simulink model "Compare_Simscape_Simulink"  (R2023a)
settings: Solver=VariableStepAuto  StartTime=0.0  StopTime=10  RelTol=1e-3
model workspace (MAT data in the model file):
  Ks = 16000
  Kt = 190000
  Mb = 300
  Mb_max = 0.00266666666667
  Mb_min = 0.00392156862745
  Mw = 60
  Mw_max = 63
  Mw_min = 57
  bs_max = 1350
  bs_min = 650
  ks_max = 20800
  ks_min = 11200
  kt_max = 209000
  kt_min = 171000
values from neighbouring files (symbols this model uses):
  Ac = (inv(value(N)))*(value(A_hat) - value(Y)*A*value(X)-value(N)*Bc*C1*value(X)-value(Y)*B1*Cc*value(M)')*(inv(value(M)'))    [Active_suspension_output_FB.m]
  Bc = (inv(value(N)))* value(B_hat)    [Active_suspension_output_FB.m]
  bs = 1000    [Active_suspension_output_FB.m]
  Cc = value(C_hat)*(inv(value(M)'))    [Active_suspension_output_FB.m]
  ks = 16000    [Active_suspension_output_FB.m]
undefined symbols (not defined in the file or in its folder): K
libraries: fl_lib x22, nesl_utility x19, slpidlib x2, sdl_lib x2, spsStairGeneratorLib x1
settings Model: Creator=poke  LastModifiedBy=poke
settings OptimizationCC: ReuseModelBlockBuffer=off

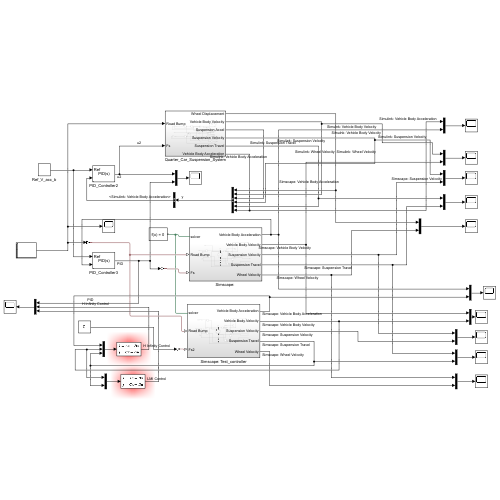
[thumbnail: Simulink's stored preview of the top-level diagram]
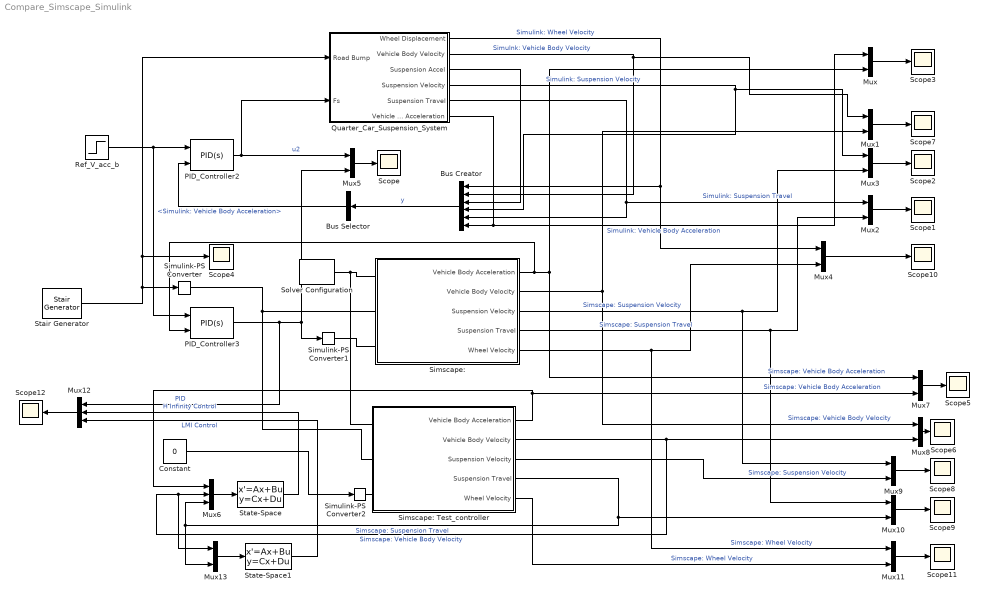
== system Compare_Simscape_Simulink ==
  Bus Creator : BusCreator  Inputs=6
  Bus Selector : BusSelector  OutputSignals=Simulink: Vehicle Body Acceleration
  Constant : Constant  Value=0
  Mux{,1..5,7..11,13} (12 alike) : Mux  Inputs=2
  Mux12 : Mux  Inputs=3
  Mux6 : Mux  Inputs=3
  PID_Controller2 : slpidlib/PID Controller (2DOF)  Controller=PID  Form=Parallel  TimeDomain=Continuous-time  UseExternalTs=off  SampleTime=-1  IntegratorMethod=Forward Euler  FilterMethod=Forward Euler  ControllerParametersSource=internal  P=10738.4637303228  I=251871.072818037  UseKiTs=off  D=98.7205538071968  N=3940.78612428139  UseFilter=on  b=0.0124821033791995  c=1.67293570854955e-05  TunerSelectOption=Transfer Function Based (PID Tuner App)  InitialConditionSource=internal  InitialConditionForIntegrator=0  InitialConditionForFilter=0  DifferentiatorICPrevScaledInput=0  ExternalReset=none  TrackingMode=off  Kt=1  LimitOutput=off  SatLimitsSource=internal  UpperSaturationLimit=inf  LowerSaturationLimit=-inf  LinearizeAsGain=on  AntiWindupMode=none  Kb=1  LimitIntegrator=off  UpperIntegratorSaturationLimit=inf  LowerIntegratorSaturationLimit=-inf  POutMin=[]  POutMax=[]  IOutMin=[]  IOutMax=[]  DOutMin=[]  DOutMax=[]  NOutMin=[]  NOutMax=[]  bOutMin=[]  bOutMax=[]  cOutMin=[]  cOutMax=[]  SumOutMin=[]  SumOutMax=[]  SaturationOutMin=[]  SaturationOutMax=[]  PParamMin=[]  PParamMax=[]  IParamMin=[]  IParamMax=[]  DParamMin=[]  DParamMax=[]  NParamMin=[]  NParamMax=[]  bParamMin=[]  bParamMax=[]  cParamMin=[]  cParamMax=[]  KbParamMin=[]  KbParamMax=[]  KtParamMin=[]  KtParamMax=[]  KbOutMin=[]  KbOutMax=[]  KtOutMin=[]  KtOutMax=[]  IntegratorOutMin=[]  IntegratorOutMax=[]  FilterOutMin=[]  FilterOutMax=[]  SumI1OutMin=[]  SumI1OutMax=[]  SumI2OutMin=[]  SumI2OutMax=[]  SumI3OutMin=[]  SumI3OutMax=[]  SumI4OutMin=[]  SumI4OutMax=[]  SumDOutMin=[]  SumDOutMax=[]  Sum1OutMin=[]  Sum1OutMax=[]  Sum2OutMin=[]  Sum2OutMax=[]  Sum3OutMin=[]  Sum3OutMax=[]  DifferentiatorOutMin=[]  DifferentiatorOutMax=[]  FilterDiffOutCoefMin=[]  FilterDiffOutCoefMax=[]  ReciprocalOutMin=[]  ReciprocalOutMax=[]  SumDenOutMin=[]  SumDenOutMax=[]  SumNumOutMin=[]  SumNumOutMax=[]  DivideOutMin=[]  DivideOutMax=[]  UdiffTsProdOutMin=[]  UdiffTsProdOutMax=[]  NTsProdOutMin=[]  NTsProdOutMax=[]  UintegralTsProdOutMin=[]  UintegralTsProdOutMax=[]  UngainTsProdOutMin=[]  UngainTsProdOutMax=[]  ClampingZeroOutDataTypeStr=Inherit: Inherit via back propagation  ClampingZeroOutMin=[]  ClampingZeroOutMax=[]  FilterDenConstantOutDataTypeStr=Inherit: Inherit via back propagation  FilterDenConstantOutMin=[]  FilterDenConstantOutMax=[]  PCopyOutDataTypeStr=Inherit: Inherit via back propagation  PCopyOutMin=[]  PCopyOutMax=[]  NCopyOutDataTypeStr=Inherit: Inherit via back propagation  NCopyOutMin=[]  NCopyOutMax=[]  IntegratorContinuousStateAttributes=''  IntegratorStateMustResolveToSignalObject=off  IntegratorRTWStateStorageClass=Auto  FilterContinuousStateAttributes=''  FilterStateMustResolveToSignalObject=off  FilterRTWStateStorageClass=Auto  ParallelPVariant=InternalParameters  IdealPVariant=Disabled  IVariant=InternalParameters  DVariant=InternalParameters  bVariant=InternalParameters  cVariant=InternalParameters  IntegratorVariant=Continuous  SatVariant=Disabled  AWVariant=Passthrough  PCopyVariant=Disabled  TRVariant=Disabled  FdbkBlocksVariant=Forward  IdealPFdbkVariant=Disabled  SatFdbkVariant=Disabled  DerivativeFilterVariant=ContFilter  NVariant=InternalParameters  NCopyVariant=Disabled  FilterICVariant=InternalICsFilter  IntegratorICVariant=InternalICs  ExternalResetVariant=Disabled  TRSumVariant=Passthrough  SumFdbkVariant=Disabled  SumVariant=Sum_PID  TsampFilterVariant=InternalTs  TsampNgainVariant=Passthrough  TsampIntegralVariant=Disabled_SignalSpec  ExternalSaturationOutDataTypeStr=Inherit: Same as second input
  PID_Controller3 : slpidlib/PID Controller (2DOF)  Controller=PID  Form=Parallel  TimeDomain=Continuous-time  UseExternalTs=off  SampleTime=-1  IntegratorMethod=Forward Euler  FilterMethod=Forward Euler  ControllerParametersSource=internal  P=10738.4637303228  I=251871.072818037  UseKiTs=off  D=98.7205538071968  N=3940.78612428139  UseFilter=on  b=0.0124821033791995  c=1.67293570854955e-05  TunerSelectOption=Transfer Function Based (PID Tuner App)  InitialConditionSource=internal  InitialConditionForIntegrator=0  InitialConditionForFilter=0  DifferentiatorICPrevScaledInput=0  ExternalReset=none  TrackingMode=off  Kt=1  LimitOutput=off  SatLimitsSource=internal  UpperSaturationLimit=inf  LowerSaturationLimit=-inf  LinearizeAsGain=on  AntiWindupMode=none  Kb=1  LimitIntegrator=off  UpperIntegratorSaturationLimit=inf  LowerIntegratorSaturationLimit=-inf  POutMin=[]  POutMax=[]  IOutMin=[]  IOutMax=[]  DOutMin=[]  DOutMax=[]  NOutMin=[]  NOutMax=[]  bOutMin=[]  bOutMax=[]  cOutMin=[]  cOutMax=[]  SumOutMin=[]  SumOutMax=[]  SaturationOutMin=[]  SaturationOutMax=[]  PParamMin=[]  PParamMax=[]  IParamMin=[]  IParamMax=[]  DParamMin=[]  DParamMax=[]  NParamMin=[]  NParamMax=[]  bParamMin=[]  bParamMax=[]  cParamMin=[]  cParamMax=[]  KbParamMin=[]  KbParamMax=[]  KtParamMin=[]  KtParamMax=[]  KbOutMin=[]  KbOutMax=[]  KtOutMin=[]  KtOutMax=[]  IntegratorOutMin=[]  IntegratorOutMax=[]  FilterOutMin=[]  FilterOutMax=[]  SumI1OutMin=[]  SumI1OutMax=[]  SumI2OutMin=[]  SumI2OutMax=[]  SumI3OutMin=[]  SumI3OutMax=[]  SumI4OutMin=[]  SumI4OutMax=[]  SumDOutMin=[]  SumDOutMax=[]  Sum1OutMin=[]  Sum1OutMax=[]  Sum2OutMin=[]  Sum2OutMax=[]  Sum3OutMin=[]  Sum3OutMax=[]  DifferentiatorOutMin=[]  DifferentiatorOutMax=[]  FilterDiffOutCoefMin=[]  FilterDiffOutCoefMax=[]  ReciprocalOutMin=[]  ReciprocalOutMax=[]  SumDenOutMin=[]  SumDenOutMax=[]  SumNumOutMin=[]  SumNumOutMax=[]  DivideOutMin=[]  DivideOutMax=[]  UdiffTsProdOutMin=[]  UdiffTsProdOutMax=[]  NTsProdOutMin=[]  NTsProdOutMax=[]  UintegralTsProdOutMin=[]  UintegralTsProdOutMax=[]  UngainTsProdOutMin=[]  UngainTsProdOutMax=[]  ClampingZeroOutDataTypeStr=Inherit: Inherit via back propagation  ClampingZeroOutMin=[]  ClampingZeroOutMax=[]  FilterDenConstantOutDataTypeStr=Inherit: Inherit via back propagation  FilterDenConstantOutMin=[]  FilterDenConstantOutMax=[]  PCopyOutDataTypeStr=Inherit: Inherit via back propagation  PCopyOutMin=[]  PCopyOutMax=[]  NCopyOutDataTypeStr=Inherit: Inherit via back propagation  NCopyOutMin=[]  NCopyOutMax=[]  IntegratorContinuousStateAttributes=''  IntegratorStateMustResolveToSignalObject=off  IntegratorRTWStateStorageClass=Auto  FilterContinuousStateAttributes=''  FilterStateMustResolveToSignalObject=off  FilterRTWStateStorageClass=Auto  ParallelPVariant=InternalParameters  IdealPVariant=Disabled  IVariant=InternalParameters  DVariant=InternalParameters  bVariant=InternalParameters  cVariant=InternalParameters  IntegratorVariant=Continuous  SatVariant=Disabled  AWVariant=Passthrough  PCopyVariant=Disabled  TRVariant=Disabled  FdbkBlocksVariant=Forward  IdealPFdbkVariant=Disabled  SatFdbkVariant=Disabled  DerivativeFilterVariant=ContFilter  NVariant=InternalParameters  NCopyVariant=Disabled  FilterICVariant=InternalICsFilter  IntegratorICVariant=InternalICs  ExternalResetVariant=Disabled  TRSumVariant=Passthrough  SumFdbkVariant=Disabled  SumVariant=Sum_PID  TsampFilterVariant=InternalTs  TsampNgainVariant=Passthrough  TsampIntegralVariant=Disabled_SignalSpec  ExternalSaturationOutDataTypeStr=Inherit: Same as second input
  Quarter_Car_Suspension_System : Subsystem
  Ref_V_acc_b : Step  After=0  SampleTime=0
  Scope{,1..12} (13 alike) : Scope
  "Simscape: " : Subsystem
  Simscape: Test_controller : Subsystem
  Simulink-PS Converter : nesl_utility/Simulink-PS Converter  PhysicalDomain=network_engine_domain  SubClassName=ps_input  LeftPortType=input  RightPortType=output  PseudoPeriodic=off  Frequencies=[]  NoiseDistribution=none  NoiseParameters=[]  Unit=1  AffineConversion=off  FilteringAndDerivatives=provide  SimscapeFilterOrder=1  InputFilterTimeConstant=0.001  UdotUserProvided=0
  Simulink-PS Converter1 : nesl_utility/Simulink-PS Converter  PhysicalDomain=network_engine_domain  SubClassName=ps_input  LeftPortType=input  RightPortType=output  PseudoPeriodic=off  Frequencies=[]  NoiseDistribution=none  NoiseParameters=[]  Unit=1  AffineConversion=off  FilteringAndDerivatives=provide  SimscapeFilterOrder=1  InputFilterTimeConstant=0.001  UdotUserProvided=0
  Simulink-PS Converter2 : nesl_utility/Simulink-PS Converter  PhysicalDomain=network_engine_domain  SubClassName=ps_input  LeftPortType=input  RightPortType=output  PseudoPeriodic=off  Frequencies=[]  NoiseDistribution=none  NoiseParameters=[]  Unit=1  AffineConversion=off  FilteringAndDerivatives=provide  SimscapeFilterOrder=1  InputFilterTimeConstant=0.001  UdotUserProvided=0
  Solver Configuration : nesl_utility/Solver Configuration  PhysicalDomain=network_engine_domain  SubClassName=solver  LeftPortType=input  RightPortType=generic  Tones=[]  Harmonics=[]  SimulateNoise=off  Profile=off  UseLocalSampling=off  EnableSwitchedLinearOptims=on  FrequencyDomain=off  UseCCode=off  RelTol=0.001  AbsTol=0.001  MinStep=1e-09  ToWorkspace=off  RevertToSquareIcSolve=off  NumHomotopyIterations=100  PhasorMode=off  PhasorModeNumHarmonics=1  ConsistencySolver=NEWTON_XTOL_AFTER_FTOL  IndexReductionMethod=DerivativeReplacement  DoDC=off  ResidualTolerance=1e-09  ConsistencyTolSource=GLOBAL  ConsistencyAbsTol=0.001  ConsistencyRelTol=0.001  ConsistencyTolFactor=0.001  UseLocalSolver=off  LocalSolverChoice=NE_BACKWARD_EULER_ADVANCER  ResolveIndetEquations=on  FunctionEvalNumThread=1  LocalSolverSampleTime=0.001  DoFixedCost=off  MaxNonlinIter=3  MaxModeIter=2  ComputeImpulses=off  ImpulseIterations=2  LinearAlgebra=auto  LinearAlgebraNumThread=0  EquationFormulation=NE_TIME_EF  DelaysMemoryBudget=1024  AutomaticFiltering=on  FilteringTimeConstant=0.001  PartitionStorageMethod=AS_NEEDED  PartitionMemoryBudget=1024  PartitionMethod=ROBUST
  Stair Generator : spsStairGeneratorLib/Stair Generator  t=t  e=roaddist  Ts=0
  State-Space : StateSpace  A=K.A  B=K.B  C=K.C  D=K.D  InitialCondition=0
  State-Space1 : StateSpace  A=Ac  B=Bc  C=Cc  D=[0 0]  InitialCondition=0
  wires:
  Quarter_Car_Suspension_System/6(Vehicle Body Acceleration) -> Mux/1, Bus Creator/6  "Simulink: Vehicle Body Acceleration"
  Quarter_Car_Suspension_System/4(Suspension Velocity) -> Bus Creator/4, Mux3/1  "Simulink: Suspension Velocity"
  Quarter_Car_Suspension_System/1(Wheel Displacement) -> Bus Creator/1, Mux4/1  "Simulink: Wheel Velocity"
  Quarter_Car_Suspension_System/2(Vehicle Body Velocity) -> Bus Creator/2, Mux1/1  "Simulnk: Vehicle Body Velocity"
  Mux/1 -> Scope3/1
  Mux1/1 -> Scope7/1
  Quarter_Car_Suspension_System/5(Suspension Travel) -> Bus Creator/5, Mux2/1  "Simulink: Suspension Travel"
  Mux2/1 -> Scope1/1
  Mux3/1 -> Scope2/1
  Mux4/1 -> Scope10/1
  "Simscape: "/1(Vehicle Body Acceleration) -> PID_Controller3/2, Mux7/1, Mux/2  "Simscape: Vehicle Body Acceleration"
  "Simscape: "/2(Vehicle Body Velocity) -> Mux8/1, Mux1/2  "Simscape: Vehicle Body Velocity"
  "Simscape: "/3(Suspension Velocity) -> Mux9/1, Mux3/2  "Simscape: Suspension Velocity"
  "Simscape: "/4(Suspension Travel) -> Mux10/1, Mux2/2  "Simscape: Suspension Travel"
  "Simscape: "/5(Wheel Velocity) -> Mux11/1, Mux4/2  "Simscape: Wheel Velocity"
  PID_Controller2/1 -> Mux5/1, Quarter_Car_Suspension_System/2(Fs)  "u2"
  Bus Selector/1 -> PID_Controller2/2  "<Simulink: Vehicle Body Acceleration>"
  Bus Creator/1 -> Bus Selector/1  "y"
  Ref_V_acc_b/1 -> PID_Controller3/1, PID_Controller2/1
  Quarter_Car_Suspension_System/3(Suspension Accel) -> Bus Creator/3
  Stair Generator/1 -> Scope4/1, Quarter_Car_Suspension_System/1(Road Bump), Simulink-PS Converter/1
  PID_Controller3/1 -> Mux12/1, Simulink-PS Converter1/1, Mux5/2  "PID"
  Mux5/1 -> Scope/1
  State-Space/1 -> Mux12/2  "H Infinity Control"
  Mux6/1 -> State-Space/1
  Simscape: Test_controller/1(Vehicle Body Acceleration) -> Mux7/2, Mux6/1  "Simscape: Vehicle Body Acceleration"
  Simscape: Test_controller/2(Vehicle Body Velocity) -> Mux8/2, Mux13/1, Mux6/2  "Simscape: Vehicle Body Velocity"
  Simscape: Test_controller/5(Wheel Velocity) -> Mux11/2  "Simscape: Wheel Velocity"
  Mux7/1 -> Scope5/1
  Mux8/1 -> Scope6/1
  Mux9/1 -> Scope8/1
  Simscape: Test_controller/3(Suspension Velocity) -> Mux9/2  "Simscape: Suspension Velocity"
  Mux10/1 -> Scope9/1
  Simscape: Test_controller/4(Suspension Travel) -> Mux6/3, Mux13/2, Mux10/2  "Simscape: Suspension Travel"
  Mux11/1 -> Scope11/1
  Mux12/1 -> Scope12/1
  Mux13/1 -> State-Space1/1
  State-Space1/1 -> Mux12/3  "LMI Control"
  Constant/1 -> Simulink-PS Converter2/1
  connections:
  Simulink-PS Converter/RConn1 -- Simscape: Test_controller/LConn2 -- "Simscape: "/LConn2
  Simulink-PS Converter1/RConn1 -- "Simscape: "/LConn3
  Simulink-PS Converter2/RConn1 -- Simscape: Test_controller/LConn3
  Solver Configuration/RConn1 -- Simscape: Test_controller/LConn1 -- "Simscape: "/LConn1

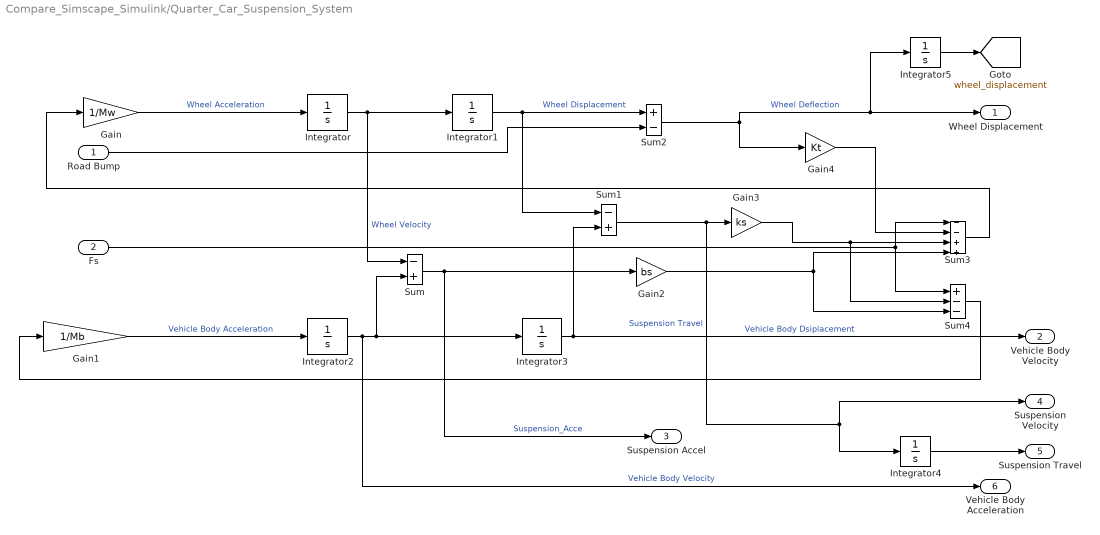
== system Compare_Simscape_Simulink/Quarter_Car_Suspension_System ==
  Road Bump : Inport
  Fs : Inport  Port=2
  Gain : Gain  Gain=1/Mw  ParamMin=1/Mw_max  ParamMax=1/Mw_min
  Gain1 : Gain  Gain=1/Mb  ParamMin=Mb_max  ParamMax=Mb_min
  Gain2 : Gain  Gain=bs  ParamMin=bs_min  ParamMax=bs_max
  Gain3 : Gain  Gain=ks  ParamMin=ks_min  ParamMax=ks_max
  Gain4 : Gain  Gain=Kt  ParamMin=kt_min  ParamMax=kt_max
  Integrator{,1..5} (6 alike) : Integrator
  Sum : Sum  Inputs=-+
  Sum1 : Sum  Inputs=-+
  Sum2 : Sum  Inputs=+-
  Sum3 : Sum  Inputs=--++
  Sum4 : Sum  Inputs=+--
  Wheel Displacement : Outport
  Vehicle Body Velocity : Outport  Port=2
  Suspension Accel : Outport  Port=3
  Suspension Velocity : Outport  Port=4
  Suspension Travel : Outport  Port=5
  Vehicle Body Acceleration : Outport  Port=6
  tag scope: wheel_displacement=global
  wires:
  Gain/1 -> Integrator/1  "Wheel Acceleration"
  Gain2/1 -> Sum4/3, Sum3/4
  Sum4/1 -> Gain1/1
  Gain1/1 -> Integrator2/1  "Vehicle Body Acceleration"
  Sum2/1 -> Gain4/1, Integrator5/1, Wheel Displacement/1  "Wheel Deflection"
  Sum3/1 -> Gain/1
  Sum/1 -> Suspension Accel/1, Gain2/1  "Suspension_Acce"
  Integrator2/1 -> Vehicle Body Acceleration/1, Integrator3/1, Sum/2  "Vehicle Body Velocity"
  Integrator1/1 -> Sum2/1, Sum1/1  "Wheel Displacement"
  Integrator3/1 -> Vehicle Body Velocity/1, Sum1/2  "Vehicle Body Dsiplacement"
  Integrator/1 -> Integrator1/1, Sum/1  "Wheel Velocity"
  Gain3/1 -> Sum4/2, Sum3/3
  Road Bump/1 -> Sum2/2
  Sum1/1 -> Suspension Velocity/1, Integrator4/1, Gain3/1  "Suspension Travel"
  Gain4/1 -> Sum3/2
  Integrator4/1 -> Suspension Travel/1
  Integrator5/1 -> [wheel_displacement]
  Fs/1 -> Sum4/1, Sum3/1

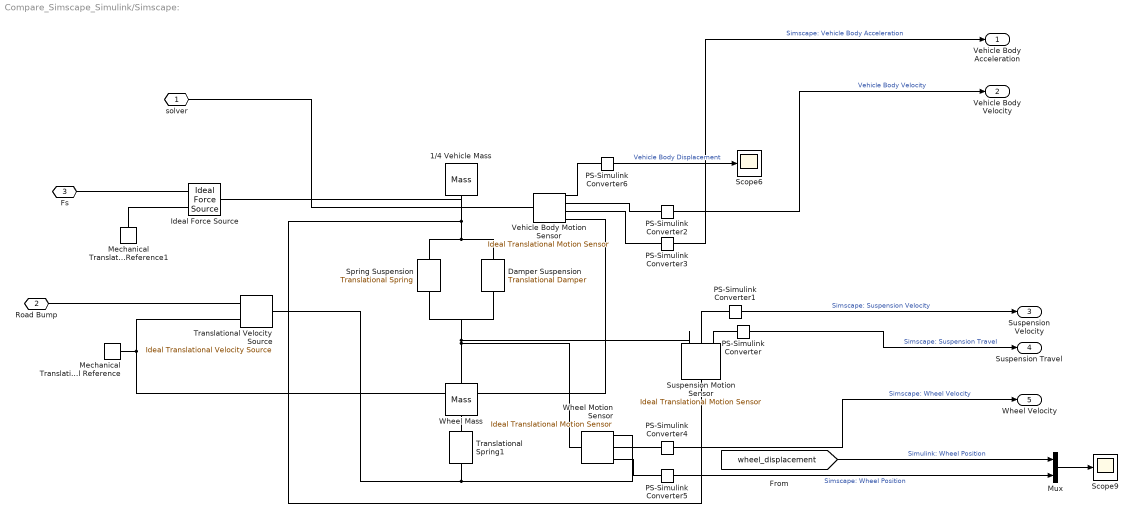
== system Compare_Simscape_Simulink/Simscape:  ==
  1/4 Vehicle Mass : fl_lib/Mechanical/Translational Elements/Mass  mass=Mb kg  num_ports=foundation.enum.numPorts2.one  v_specify=off  v_priority=High  v=0 m/s  v_nominal_specify=off  v_nominal_unit=m/s  v_nominal_value=1  f_specify=off  f_priority=None  f=0 N  f_nominal_specify=off  f_nominal_unit=N  f_nominal_value=1
  Damper Suspension : sdl_lib/Couplings & Drives/Springs & Dampers/Translational Damper  D=bs N*s/m  enable_faults=simscape.enum.onoff.off  b_fault=1e6 N*s/m  temporal_fault=simscape.enum.onoff.off  fault_time=5 s  shock_fault=simscape.enum.onoff.off  acceleration_limit=100 m/s^2  shock_limit=1  report_fault=simscape.enum.assert.action.none  thermal_port=simscape.enum.thermaleffects.omit  thermal_mass=50 kJ/K  temperature_specify=off  temperature_priority=High  temperature=300 K  temperature_nominal_specify=off  temperature_nominal_unit=K  temperature_nominal_value=1
  Ideal Force Source : fl_lib/Mechanical/Mechanical Sources/Ideal Force Source
  Mechanical Translational Reference : fl_lib/Mechanical/Translational Elements/Mechanical Translational Reference
  Mechanical Translational Reference1 : fl_lib/Mechanical/Translational Elements/Mechanical Translational Reference
  Mux : Mux  Inputs=2
  PS-Simulink Converter{,1,4..5} (4 alike) : nesl_utility/PS-Simulink Converter  PhysicalDomain=network_engine_domain  SubClassName=ps_output  LeftPortType=input  RightPortType=output  PseudoPeriodic=off  Frequencies=[]  VectorFormat=inherit  Unit=inherit  AffineConversion=off
  PS-Simulink Converter2 : nesl_utility/PS-Simulink Converter  PhysicalDomain=network_engine_domain  SubClassName=ps_output  LeftPortType=input  RightPortType=output  PseudoPeriodic=off  Frequencies=[]  VectorFormat=inherit  Unit=inherit  AffineConversion=on
  PS-Simulink Converter3 : nesl_utility/PS-Simulink Converter  PhysicalDomain=network_engine_domain  SubClassName=ps_output  LeftPortType=input  RightPortType=output  PseudoPeriodic=off  Frequencies=[]  VectorFormat=inherit  Unit=inherit  AffineConversion=on
  PS-Simulink Converter6 : nesl_utility/PS-Simulink Converter  PhysicalDomain=network_engine_domain  SubClassName=ps_output  LeftPortType=input  RightPortType=output  PseudoPeriodic=off  Frequencies=[]  VectorFormat=inherit  Unit=inherit  AffineConversion=on
  Scope6 : Scope
  Scope9 : Scope
  Spring Suspension : fl_lib/Mechanical/Translational Elements/Translational Spring  spr_rate=Ks N/m  v_specify=off  v_priority=None  v=0 m/s  v_nominal_specify=off  v_nominal_unit=m/s  v_nominal_value=1  f_specify=off  f_priority=None  f=0 N  f_nominal_specify=off  f_nominal_unit=N  f_nominal_value=1  x_specify=off  x_priority=High  x=0 m  x_nominal_specify=off  x_nominal_unit=m  x_nominal_value=1
  Suspension Motion Sensor : fl_lib/Mechanical/Mechanical Sensors/Ideal Translational Motion Sensor  reference=foundation.enum.MeasurementReference.difference  acceleration_port=false  velocity_port=true  position_port=true  offset=0 m
  Translational Velocity Source : fl_lib/Mechanical/Mechanical Sources/Ideal Translational Velocity Source
  Translational Spring1 : fl_lib/Mechanical/Translational Elements/Translational Spring  spr_rate=Kt N/m  v_specify=off  v_priority=None  v=0 m/s  v_nominal_specify=off  v_nominal_unit=m/s  v_nominal_value=1  f_specify=off  f_priority=None  f=0 N  f_nominal_specify=off  f_nominal_unit=N  f_nominal_value=1  x_specify=off  x_priority=High  x=0 m  x_nominal_specify=off  x_nominal_unit=m  x_nominal_value=1
  Vehicle Body Motion Sensor : fl_lib/Mechanical/Mechanical Sensors/Ideal Translational Motion Sensor  reference=foundation.enum.MeasurementReference.difference  acceleration_port=true  velocity_port=true  position_port=true  offset=0 m
      settings: InternalSimscapePortConfiguration="{\"Bottom\":[],\"Left\":[{\"id\":\"R\",\"label\":\"R\",\"type\":\"foundation.mechanical.translational.translational\"}],\"Right\":[{\"id\":\"C\",\"label\":\"C\",\"type\":\"foundation.mechanical.translational.translational\"},{\"id\":\"A\",\"label\":\"A\",\"type\":\"output\"},{\"id\":\"V\",\"label\":\"V\",\"type\":\"output\"},{\"id\":\"P\",\"label\":\"P\",\"type\":\"output\"}],\"Top\":[]}"
  Wheel Motion Sensor : fl_lib/Mechanical/Mechanical Sensors/Ideal Translational Motion Sensor  reference=foundation.enum.MeasurementReference.difference  acceleration_port=false  velocity_port=true  position_port=true  offset=0 m
  Wheel Mass : fl_lib/Mechanical/Translational Elements/Mass  mass=Mw kg  num_ports=foundation.enum.numPorts2.two  v_specify=off  v_priority=High  v=0 m/s  v_nominal_specify=off  v_nominal_unit=m/s  v_nominal_value=1  f_specify=off  f_priority=None  f=0 N  f_nominal_specify=off  f_nominal_unit=N  f_nominal_value=1
      settings: InternalSimscapePortConfiguration="{\"Bottom\":[],\"Left\":[{\"id\":\"M\",\"label\":\"\",\"type\":\"foundation.mechanical.translational.translational\"}],\"Right\":[{\"id\":\"N\",\"label\":\"\",\"type\":\"foundation.mechanical.translational.translational\"}],\"Top\":[]}"
  solver : PMIOPort  Side=Left
  Road Bump : PMIOPort  Port=2  Side=Left
  Fs : PMIOPort  Port=3  Side=Left
  Vehicle Body Acceleration : Outport
  Vehicle Body Velocity : Outport  Port=2
  Suspension Velocity : Outport  Port=3
  Suspension Travel : Outport  Port=4
  Wheel Velocity : Outport  Port=5
  wires:
  PS-Simulink Converter3/1 -> Vehicle Body Acceleration/1  "Simscape: Vehicle Body Acceleration"
  PS-Simulink Converter/1 -> Suspension Travel/1  "Simscape: Suspension Travel"
  PS-Simulink Converter4/1 -> Wheel Velocity/1  "Simscape: Wheel Velocity"
  PS-Simulink Converter6/1 -> Scope6/1  "Vehicle Body Displacement"
  PS-Simulink Converter2/1 -> Vehicle Body Velocity/1  "Vehicle Body Velocity"
  PS-Simulink Converter1/1 -> Suspension Velocity/1  "Simscape: Suspension Velocity"
  Mux/1 -> Scope9/1
  PS-Simulink Converter5/1 -> Mux/2  "Simscape: Wheel Position"
  [wheel_displacement] -> Mux/1  "Simulink: Wheel Position"
  connections:
  PS-Simulink Converter1/LConn1 -- Suspension Motion Sensor/RConn2
  PS-Simulink Converter4/LConn1 -- Wheel Motion Sensor/RConn2
  Suspension Motion Sensor/RConn1 -- Damper Suspension/RConn1 -- Spring Suspension/RConn1 -- Wheel Motion Sensor/LConn1 -- Wheel Mass/LConn1
  Mechanical Translational Reference/LConn1 -- Translational Velocity Source/RConn2 -- Vehicle Body Motion Sensor/RConn1
  Vehicle Body Motion Sensor/RConn3 -- PS-Simulink Converter2/LConn1
  Spring Suspension/LConn1 -- Ideal Force Source/LConn1 -- Vehicle Body Motion Sensor/LConn1 -- solver/RConn1 -- 1/4 Vehicle Mass/LConn1 -- Suspension Motion Sensor/LConn1 -- Damper Suspension/LConn1
  Translational Velocity Source/LConn1 -- Wheel Motion Sensor/RConn1 -- Translational Spring1/RConn1
  Translational Spring1/LConn1 -- Wheel Mass/RConn1
  Wheel Motion Sensor/RConn3 -- PS-Simulink Converter5/LConn1
  Vehicle Body Motion Sensor/RConn2 -- PS-Simulink Converter3/LConn1
  PS-Simulink Converter6/LConn1 -- Vehicle Body Motion Sensor/RConn4
  Suspension Motion Sensor/RConn3 -- PS-Simulink Converter/LConn1
  Translational Velocity Source/RConn1 -- Road Bump/RConn1
  Fs/RConn1 -- Ideal Force Source/RConn1
  Mechanical Translational Reference1/LConn1 -- Ideal Force Source/RConn2

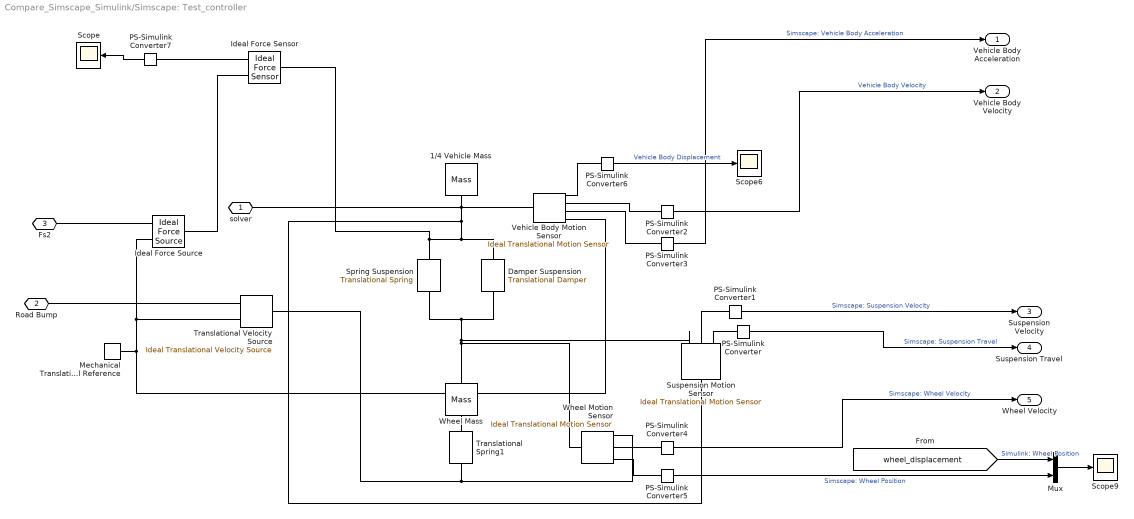
== system Compare_Simscape_Simulink/Simscape: Test_controller ==
  1/4 Vehicle Mass : fl_lib/Mechanical/Translational Elements/Mass  mass=Mb kg  num_ports=foundation.enum.numPorts2.one  v_specify=off  v_priority=High  v=0 m/s  v_nominal_specify=off  v_nominal_unit=m/s  v_nominal_value=1  f_specify=off  f_priority=None  f=0 N  f_nominal_specify=off  f_nominal_unit=N  f_nominal_value=1
  Damper Suspension : sdl_lib/Couplings & Drives/Springs & Dampers/Translational Damper  D=bs N*s/m  enable_faults=simscape.enum.onoff.off  b_fault=1e6 N*s/m  temporal_fault=simscape.enum.onoff.off  fault_time=5 s  shock_fault=simscape.enum.onoff.off  acceleration_limit=100 m/s^2  shock_limit=1  report_fault=simscape.enum.assert.action.none  thermal_port=simscape.enum.thermaleffects.omit  thermal_mass=50 kJ/K  temperature_specify=off  temperature_priority=High  temperature=300 K  temperature_nominal_specify=off  temperature_nominal_unit=K  temperature_nominal_value=1
  Ideal Force Sensor : fl_lib/Mechanical/Mechanical Sensors/Ideal Force Sensor
  Ideal Force Source : fl_lib/Mechanical/Mechanical Sources/Ideal Force Source
  Mechanical Translational Reference : fl_lib/Mechanical/Translational Elements/Mechanical Translational Reference
  Mux : Mux  Inputs=2
  PS-Simulink Converter{,1,4..5,7} (5 alike) : nesl_utility/PS-Simulink Converter  PhysicalDomain=network_engine_domain  SubClassName=ps_output  LeftPortType=input  RightPortType=output  PseudoPeriodic=off  Frequencies=[]  VectorFormat=inherit  Unit=inherit  AffineConversion=off
  PS-Simulink Converter2 : nesl_utility/PS-Simulink Converter  PhysicalDomain=network_engine_domain  SubClassName=ps_output  LeftPortType=input  RightPortType=output  PseudoPeriodic=off  Frequencies=[]  VectorFormat=inherit  Unit=inherit  AffineConversion=on
  PS-Simulink Converter3 : nesl_utility/PS-Simulink Converter  PhysicalDomain=network_engine_domain  SubClassName=ps_output  LeftPortType=input  RightPortType=output  PseudoPeriodic=off  Frequencies=[]  VectorFormat=inherit  Unit=inherit  AffineConversion=on
  PS-Simulink Converter6 : nesl_utility/PS-Simulink Converter  PhysicalDomain=network_engine_domain  SubClassName=ps_output  LeftPortType=input  RightPortType=output  PseudoPeriodic=off  Frequencies=[]  VectorFormat=inherit  Unit=inherit  AffineConversion=on
  Scope : Scope
  Scope6 : Scope
  Scope9 : Scope
  Spring Suspension : fl_lib/Mechanical/Translational Elements/Translational Spring  spr_rate=Ks N/m  v_specify=off  v_priority=None  v=0 m/s  v_nominal_specify=off  v_nominal_unit=m/s  v_nominal_value=1  f_specify=off  f_priority=None  f=0 N  f_nominal_specify=off  f_nominal_unit=N  f_nominal_value=1  x_specify=off  x_priority=High  x=0 m  x_nominal_specify=off  x_nominal_unit=m  x_nominal_value=1
  Suspension Motion Sensor : fl_lib/Mechanical/Mechanical Sensors/Ideal Translational Motion Sensor  reference=foundation.enum.MeasurementReference.difference  acceleration_port=false  velocity_port=true  position_port=true  offset=0 m
  Translational Velocity Source : fl_lib/Mechanical/Mechanical Sources/Ideal Translational Velocity Source
  Translational Spring1 : fl_lib/Mechanical/Translational Elements/Translational Spring  spr_rate=Kt N/m  v_specify=off  v_priority=None  v=0 m/s  v_nominal_specify=off  v_nominal_unit=m/s  v_nominal_value=1  f_specify=off  f_priority=None  f=0 N  f_nominal_specify=off  f_nominal_unit=N  f_nominal_value=1  x_specify=off  x_priority=High  x=0 m  x_nominal_specify=off  x_nominal_unit=m  x_nominal_value=1
  Vehicle Body Motion Sensor : fl_lib/Mechanical/Mechanical Sensors/Ideal Translational Motion Sensor  reference=foundation.enum.MeasurementReference.difference  acceleration_port=true  velocity_port=true  position_port=true  offset=0 m
      settings: InternalSimscapePortConfiguration="{\"Bottom\":[],\"Left\":[{\"id\":\"R\",\"label\":\"R\",\"type\":\"foundation.mechanical.translational.translational\"}],\"Right\":[{\"id\":\"C\",\"label\":\"C\",\"type\":\"foundation.mechanical.translational.translational\"},{\"id\":\"A\",\"label\":\"A\",\"type\":\"output\"},{\"id\":\"V\",\"label\":\"V\",\"type\":\"output\"},{\"id\":\"P\",\"label\":\"P\",\"type\":\"output\"}],\"Top\":[]}"
  Wheel Motion Sensor : fl_lib/Mechanical/Mechanical Sensors/Ideal Translational Motion Sensor  reference=foundation.enum.MeasurementReference.difference  acceleration_port=false  velocity_port=true  position_port=true  offset=0 m
  Wheel Mass : fl_lib/Mechanical/Translational Elements/Mass  mass=Mw kg  num_ports=foundation.enum.numPorts2.two  v_specify=off  v_priority=High  v=0 m/s  v_nominal_specify=off  v_nominal_unit=m/s  v_nominal_value=1  f_specify=off  f_priority=None  f=0 N  f_nominal_specify=off  f_nominal_unit=N  f_nominal_value=1
      settings: InternalSimscapePortConfiguration="{\"Bottom\":[],\"Left\":[{\"id\":\"M\",\"label\":\"\",\"type\":\"foundation.mechanical.translational.translational\"}],\"Right\":[{\"id\":\"N\",\"label\":\"\",\"type\":\"foundation.mechanical.translational.translational\"}],\"Top\":[]}"
  solver : PMIOPort  Side=Left
  Road Bump : PMIOPort  Port=2  Side=Left
  Fs2 : PMIOPort  Port=3  Side=Left
  Vehicle Body Acceleration : Outport
  Vehicle Body Velocity : Outport  Port=2
  Suspension Velocity : Outport  Port=3
  Suspension Travel : Outport  Port=4
  Wheel Velocity : Outport  Port=5
  wires:
  [wheel_displacement] -> Mux/1  "Simulink: Wheel Position"
  PS-Simulink Converter5/1 -> Mux/2  "Simscape: Wheel Position"
  Mux/1 -> Scope9/1
  PS-Simulink Converter1/1 -> Suspension Velocity/1  "Simscape: Suspension Velocity"
  PS-Simulink Converter2/1 -> Vehicle Body Velocity/1  "Vehicle Body Velocity"
  PS-Simulink Converter6/1 -> Scope6/1  "Vehicle Body Displacement"
  PS-Simulink Converter4/1 -> Wheel Velocity/1  "Simscape: Wheel Velocity"
  PS-Simulink Converter/1 -> Suspension Travel/1  "Simscape: Suspension Travel"
  PS-Simulink Converter3/1 -> Vehicle Body Acceleration/1  "Simscape: Vehicle Body Acceleration"
  PS-Simulink Converter7/1 -> Scope/1
  connections:
  Fs2/RConn1 -- Ideal Force Source/RConn1
  Translational Velocity Source/RConn1 -- Road Bump/RConn1
  Suspension Motion Sensor/RConn3 -- PS-Simulink Converter/LConn1
  PS-Simulink Converter6/LConn1 -- Vehicle Body Motion Sensor/RConn4
  Vehicle Body Motion Sensor/RConn2 -- PS-Simulink Converter3/LConn1
  Wheel Motion Sensor/RConn3 -- PS-Simulink Converter5/LConn1
  Translational Spring1/LConn1 -- Wheel Mass/RConn1
  Wheel Motion Sensor/RConn1 -- Translational Spring1/RConn1 -- Translational Velocity Source/LConn1
  Vehicle Body Motion Sensor/LConn1 -- solver/RConn1 -- 1/4 Vehicle Mass/LConn1 -- Suspension Motion Sensor/LConn1 -- Ideal Force Sensor/LConn1 -- Spring Suspension/LConn1 -- Damper Suspension/LConn1
  Vehicle Body Motion Sensor/RConn3 -- PS-Simulink Converter2/LConn1
  Mechanical Translational Reference/LConn1 -- Vehicle Body Motion Sensor/RConn1 -- Ideal Force Source/RConn2 -- Translational Velocity Source/RConn2
  Wheel Mass/LConn1 -- Wheel Motion Sensor/LConn1 -- Spring Suspension/RConn1 -- Damper Suspension/RConn1 -- Suspension Motion Sensor/RConn1
  PS-Simulink Converter4/LConn1 -- Wheel Motion Sensor/RConn2
  PS-Simulink Converter1/LConn1 -- Suspension Motion Sensor/RConn2
  PS-Simulink Converter7/LConn1 -- Ideal Force Sensor/RConn2
  Ideal Force Sensor/RConn1 -- Ideal Force Source/LConn1
